simulink model "bibli_SM_R2023b_QUEVAL_20240121"  (R2023b)
settings: Solver=VariableStepAuto  StartTime=0.0  StopTime=10  MaxStep=1e-3  RelTol=1e-3
values from neighbouring files (symbols this model uses):
  Clark = [	2/3		-1/3		-1/3 ... (first row only)    [param_EESM.m]    (also in param_EESMdampers.m; param_PMSM.m)
  Fif = 0.259*3    (= 0.777)    [param_PMSM.m]
  InvClark = inv(Clark)    [param_EESM.m]    (also in param_EESMdampers.m; param_PMSM.m)
  INVL = inv(L)    [param_EESM.m]    (also in param_EESMdampers.m)
  J = 0.5    [param_EESM.m]    (also in param_EESMdampers.m; param_PMSM.m)
  Ld = 1.59e-2    (= 0.0159)    [param_EESM.m]    (also in param_EESMdampers.m; param_PMSM.m)
  Lq = 1.59e-2    (= 0.0159)    [param_EESM.m]    (also in param_EESMdampers.m; param_PMSM.m)
  M = [     0	    0	    -1 ... (first row only)    [param_EESM.m]    (also in param_EESMdampers.m = [     0	    0	    0	    -1	    0; param_PMSM.m = [     0	    -1)
  npp = 2    [param_EESM.m]    (also in param_EESMdampers.m; param_PMSM.m)
  R = [     Rs	    0	    0 ... (first row only)    [param_EESM.m]    (also in param_EESMdampers.m = [     Rs	    0	    0	    0	    0; param_PMSM.m = [     Rs	    0)
undefined symbols (not defined in the file or in its folder): fd, iao_pd_si, ibo_pd_si, ico_pd_si, Ts
libraries: spsSeriesRLCBranchLib x9, spsControlledCurrentSourceLib x9, spsVoltageMeasurementLib x9, spsControlledVoltageSourceLib x6, spsIdealSwitchLib x6, spsDCVoltageSourceLib x1, spsGroundLib x1, spspowerguiLib x1
(part 2 of 2)

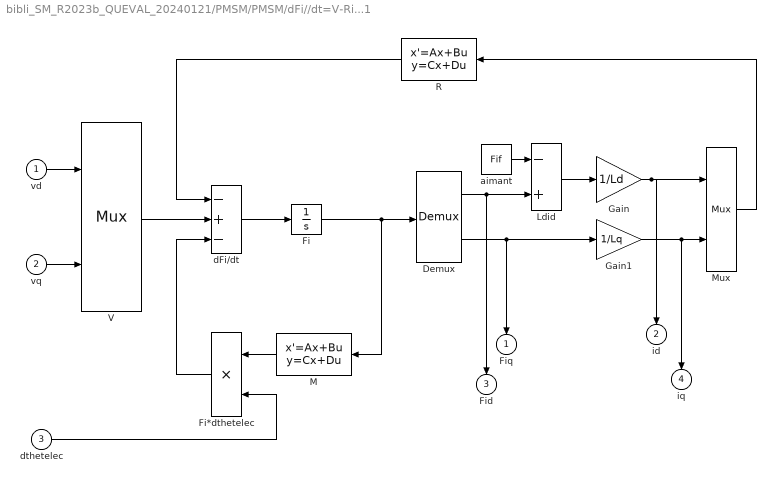
== system bibli_SM_R2023b_QUEVAL_20240121/PMSM/PMSM/dFi//dt=V-Ri...1 ==
  vd : Inport
  vq : Inport  Port=2
  dthetelec : Inport  Port=3
  Demux : Demux  Outputs=2
      settings: DisplayOption=none
  Fi : Integrator  InitialCondition=[Fif 0]
  Fi*dthetelec : Product  InputSameDT=on  SaturateOnIntegerOverflow=on  OutDataTypeStr=Inherit: Same as first input
  Gain : Gain  Gain=1/Ld  SaturateOnIntegerOverflow=on  OutDataTypeStr=Inherit: Same as input  ParamDataTypeStr=Inherit: Same as input
  Gain1 : Gain  Gain=1/Lq  SaturateOnIntegerOverflow=on  OutDataTypeStr=Inherit: Same as input  ParamDataTypeStr=Inherit: Same as input
  Ldid : Sum  Inputs=-+  InputSameDT=on  SaturateOnIntegerOverflow=on  OutDataTypeStr=Inherit: Same as first input
  M : StateSpace  A=[]  B=[]  C=[]  D=K  InitialCondition=0  mask(Matrix gain){K=M}
      mask prompts: K "Gain matrix:"
      mask help: Matrix Gain.
      mask Help: Multiplies input vector by entered matrix to produce output vector (y=Au).
      mask Display: disp('Matrice')
  Mux : Mux  Inputs=2
  R : StateSpace  A=[]  B=[]  C=[]  D=K  InitialCondition=0  mask(Matrix gain){K=R}
      mask prompts: K "Gain matrix:"
      mask help: Matrix Gain.
      mask Help: Multiplies input vector by entered matrix to produce output vector (y=Au).
      mask Display: disp('Matrice')
  V : Mux  Inputs=2
  aimant : Constant  Value=Fif
  dFi/dt : Sum  Inputs=-+-  InputSameDT=on  SaturateOnIntegerOverflow=on  OutDataTypeStr=Inherit: Same as first input
  Fiq : Outport  InitialOutput=0  VectorParamsAs1DForOutWhenUnconnected=off
  id : Outport  Port=2  InitialOutput=0  VectorParamsAs1DForOutWhenUnconnected=off
  Fid : Outport  Port=3  InitialOutput=0  VectorParamsAs1DForOutWhenUnconnected=off
  iq : Outport  Port=4  InitialOutput=0  VectorParamsAs1DForOutWhenUnconnected=off
  wires:
  Mux/1 -> R/1
  Gain1/1 -> iq/1, Mux/2
  Gain/1 -> id/1, Mux/1
  Demux/2 -> Fiq/1, Gain1/1
  Ldid/1 -> Gain/1
  aimant/1 -> Ldid/1
  Demux/1 -> Fid/1, Ldid/2
  Fi*dthetelec/1 -> dFi/dt/3
  M/1 -> Fi*dthetelec/1
  vq/1 -> V/2
  vd/1 -> V/1
  dFi/dt/1 -> Fi/1
  R/1 -> dFi/dt/1
  V/1 -> dFi/dt/2
  dthetelec/1 -> Fi*dthetelec/2
  Fi/1 -> Demux/1, M/1

== system bibli_SM_R2023b_QUEVAL_20240121/MS bobiné/MS bobiné/Park1/Clark ==
  a : Inport
  b : Inport  Port=2
  c : Inport  Port=3
  "Clark " : StateSpace  A=[]  B=[]  C=[]  D=K  InitialCondition=0  mask(Matrix Gain){K=Clark}
      mask prompts: K "Gain matrix:"
      mask help: Matrix Gain.
      mask Help: Multiplies input vector by entered matrix to produce output vector (y=Au).
      mask Display: disp('K')
  Demux : Demux  Outputs=3
      settings: DisplayOption=none
  Mux : Mux  Inputs=3
  alpha : Outport  InitialOutput=0  VectorParamsAs1DForOutWhenUnconnected=off
  beta : Outport  Port=2  InitialOutput=0  VectorParamsAs1DForOutWhenUnconnected=off
  o : Outport  Port=3  InitialOutput=0  VectorParamsAs1DForOutWhenUnconnected=off
  wires:
  Demux/3 -> o/1
  Demux/2 -> beta/1
  Demux/1 -> alpha/1
  "Clark "/1 -> Demux/1
  Mux/1 -> "Clark "/1
  c/1 -> Mux/3
  b/1 -> Mux/2
  a/1 -> Mux/1

== system bibli_SM_R2023b_QUEVAL_20240121/MS bobiné/MS bobiné/Park1/Rotation ==
  cos : Inport
  sin : Inport  Port=2
  alpha : Inport  Port=3
  beta : Inport  Port=4
  Product{,1..3} (4 alike) : Product  InputSameDT=on  RndMeth=Zero  SaturateOnIntegerOverflow=on  OutDataTypeStr=Inherit: Same as first input
  Sum : Sum  InputSameDT=on  SaturateOnIntegerOverflow=on  OutDataTypeStr=Inherit: Same as first input
  Sum1 : Sum  Inputs=-+  InputSameDT=on  SaturateOnIntegerOverflow=on  OutDataTypeStr=Inherit: Same as first input
  d : Outport  InitialOutput=0  VectorParamsAs1DForOutWhenUnconnected=off
  q : Outport  Port=2  InitialOutput=0  VectorParamsAs1DForOutWhenUnconnected=off
  wires:
  alpha/1 -> Product2/1, Product/2
  beta/1 -> Product3/2, Product1/2
  Sum1/1 -> q/1
  Sum/1 -> d/1
  Product3/1 -> Sum1/2
  Product2/1 -> Sum1/1
  cos/1 -> Product3/1, Product/1
  sin/1 -> Product2/2, Product1/1
  Product1/1 -> Sum/2
  Product/1 -> Sum/1

== system bibli_SM_R2023b_QUEVAL_20240121/MS bobiné/MS bobiné/Parkinv1/ClarkInv ==
  alpha : Inport
  beta : Inport  Port=2
  o : Inport  Port=3
  "ClarkInv " : StateSpace  A=[]  B=[]  C=[]  D=K  InitialCondition=0  mask(Matrix Gain){K=InvClark}
      mask prompts: K "Gain matrix:"
      mask help: Matrix Gain.
      mask Help: Multiplies input vector by entered matrix to produce output vector (y=Au).
      mask Display: disp('K')
  Demux : Demux  Outputs=3
      settings: DisplayOption=none
  Mux : Mux  Inputs=3
  a : Outport  InitialOutput=0  VectorParamsAs1DForOutWhenUnconnected=off
  b : Outport  Port=2  InitialOutput=0  VectorParamsAs1DForOutWhenUnconnected=off
  c : Outport  Port=3  InitialOutput=0  VectorParamsAs1DForOutWhenUnconnected=off
  wires:
  Demux/3 -> c/1
  Demux/2 -> b/1
  Demux/1 -> a/1
  "ClarkInv "/1 -> Demux/1
  Mux/1 -> "ClarkInv "/1
  o/1 -> Mux/3
  beta/1 -> Mux/2
  alpha/1 -> Mux/1

== system bibli_SM_R2023b_QUEVAL_20240121/MS bobiné/MS bobiné/Parkinv1/Rotation Inverse ==
  cos : Inport
  sin : Inport  Port=2
  d : Inport  Port=3
  q : Inport  Port=4
  Product{,1..3} (4 alike) : Product  InputSameDT=on  RndMeth=Zero  SaturateOnIntegerOverflow=on  OutDataTypeStr=Inherit: Same as first input
  Sum : Sum  Inputs=+-  InputSameDT=on  SaturateOnIntegerOverflow=on  OutDataTypeStr=Inherit: Same as first input
  Sum1 : Sum  InputSameDT=on  SaturateOnIntegerOverflow=on  OutDataTypeStr=Inherit: Same as first input
  alpha : Outport  InitialOutput=0  VectorParamsAs1DForOutWhenUnconnected=off
  beta : Outport  Port=2  InitialOutput=0  VectorParamsAs1DForOutWhenUnconnected=off
  wires:
  d/1 -> Product2/1, Product/2
  q/1 -> Product3/2, Product1/2
  Sum1/1 -> beta/1
  Sum/1 -> alpha/1
  Product3/1 -> Sum1/2
  Product2/1 -> Sum1/1
  cos/1 -> Product3/1, Product/1
  sin/1 -> Product2/2, Product1/1
  Product1/1 -> Sum/2
  Product/1 -> Sum/1

== system bibli_SM_R2023b_QUEVAL_20240121/MS bobiné amortisseurs/MS bobiné amortisseurs/Park/Clark ==
  a : Inport
  b : Inport  Port=2
  c : Inport  Port=3
  "Clark " : StateSpace  A=[]  B=[]  C=[]  D=K  InitialCondition=0  mask(Matrix Gain){K=Clark}
      mask prompts: K "Gain matrix:"
      mask help: Matrix Gain.
      mask Help: Multiplies input vector by entered matrix to produce output vector (y=Au).
      mask Display: disp('K')
  Demux : Demux  Outputs=3
      settings: DisplayOption=none
  Mux : Mux  Inputs=3
  alpha : Outport  InitialOutput=0  VectorParamsAs1DForOutWhenUnconnected=off
  beta : Outport  Port=2  InitialOutput=0  VectorParamsAs1DForOutWhenUnconnected=off
  o : Outport  Port=3  InitialOutput=0  VectorParamsAs1DForOutWhenUnconnected=off
  wires:
  Demux/3 -> o/1
  Demux/2 -> beta/1
  Demux/1 -> alpha/1
  "Clark "/1 -> Demux/1
  Mux/1 -> "Clark "/1
  c/1 -> Mux/3
  b/1 -> Mux/2
  a/1 -> Mux/1

== system bibli_SM_R2023b_QUEVAL_20240121/MS bobiné amortisseurs/MS bobiné amortisseurs/Park/Rotation ==
  cos : Inport
  sin : Inport  Port=2
  alpha : Inport  Port=3
  beta : Inport  Port=4
  Product{,1..3} (4 alike) : Product  InputSameDT=on  RndMeth=Zero  SaturateOnIntegerOverflow=on  OutDataTypeStr=Inherit: Same as first input
  Sum : Sum  InputSameDT=on  SaturateOnIntegerOverflow=on  OutDataTypeStr=Inherit: Same as first input
  Sum1 : Sum  Inputs=-+  InputSameDT=on  SaturateOnIntegerOverflow=on  OutDataTypeStr=Inherit: Same as first input
  d : Outport  InitialOutput=0  VectorParamsAs1DForOutWhenUnconnected=off
  q : Outport  Port=2  InitialOutput=0  VectorParamsAs1DForOutWhenUnconnected=off
  wires:
  alpha/1 -> Product2/1, Product/2
  beta/1 -> Product3/2, Product1/2
  Sum1/1 -> q/1
  Sum/1 -> d/1
  Product3/1 -> Sum1/2
  Product2/1 -> Sum1/1
  cos/1 -> Product3/1, Product/1
  sin/1 -> Product2/2, Product1/1
  Product1/1 -> Sum/2
  Product/1 -> Sum/1

== system bibli_SM_R2023b_QUEVAL_20240121/MS bobiné amortisseurs/MS bobiné amortisseurs/Parkinv/ClarkInv ==
  alpha : Inport
  beta : Inport  Port=2
  o : Inport  Port=3
  "ClarkInv " : StateSpace  A=[]  B=[]  C=[]  D=K  InitialCondition=0  mask(Matrix Gain){K=InvClark}
      mask prompts: K "Gain matrix:"
      mask help: Matrix Gain.
      mask Help: Multiplies input vector by entered matrix to produce output vector (y=Au).
      mask Display: disp('K')
  Demux : Demux  Outputs=3
      settings: DisplayOption=none
  Mux : Mux  Inputs=3
  a : Outport  InitialOutput=0  VectorParamsAs1DForOutWhenUnconnected=off
  b : Outport  Port=2  InitialOutput=0  VectorParamsAs1DForOutWhenUnconnected=off
  c : Outport  Port=3  InitialOutput=0  VectorParamsAs1DForOutWhenUnconnected=off
  wires:
  Demux/3 -> c/1
  Demux/2 -> b/1
  Demux/1 -> a/1
  "ClarkInv "/1 -> Demux/1
  Mux/1 -> "ClarkInv "/1
  o/1 -> Mux/3
  beta/1 -> Mux/2
  alpha/1 -> Mux/1

== system bibli_SM_R2023b_QUEVAL_20240121/MS bobiné amortisseurs/MS bobiné amortisseurs/Parkinv/Rotation Inverse ==
  cos : Inport
  sin : Inport  Port=2
  d : Inport  Port=3
  q : Inport  Port=4
  Product{,1..3} (4 alike) : Product  InputSameDT=on  RndMeth=Zero  SaturateOnIntegerOverflow=on  OutDataTypeStr=Inherit: Same as first input
  Sum : Sum  Inputs=+-  InputSameDT=on  SaturateOnIntegerOverflow=on  OutDataTypeStr=Inherit: Same as first input
  Sum1 : Sum  InputSameDT=on  SaturateOnIntegerOverflow=on  OutDataTypeStr=Inherit: Same as first input
  alpha : Outport  InitialOutput=0  VectorParamsAs1DForOutWhenUnconnected=off
  beta : Outport  Port=2  InitialOutput=0  VectorParamsAs1DForOutWhenUnconnected=off
  wires:
  d/1 -> Product2/1, Product/2
  q/1 -> Product3/2, Product1/2
  Sum1/1 -> beta/1
  Sum/1 -> alpha/1
  Product3/1 -> Sum1/2
  Product2/1 -> Sum1/1
  cos/1 -> Product3/1, Product/1
  sin/1 -> Product2/2, Product1/1
  Product1/1 -> Sum/2
  Product/1 -> Sum/1

== system bibli_SM_R2023b_QUEVAL_20240121/PMSM/PMSM/Park/Clark ==
  a : Inport
  b : Inport  Port=2
  c : Inport  Port=3
  "Clark " : StateSpace  A=[]  B=[]  C=[]  D=K  InitialCondition=0  mask(Matrix Gain){K=Clark}
      mask prompts: K "Gain matrix:"
      mask help: Matrix Gain.
      mask Help: Multiplies input vector by entered matrix to produce output vector (y=Au).
      mask Display: disp('K')
  Demux : Demux  Outputs=3
      settings: DisplayOption=none
  Mux : Mux  Inputs=3
  alpha : Outport  InitialOutput=0  VectorParamsAs1DForOutWhenUnconnected=off
  beta : Outport  Port=2  InitialOutput=0  VectorParamsAs1DForOutWhenUnconnected=off
  o : Outport  Port=3  InitialOutput=0  VectorParamsAs1DForOutWhenUnconnected=off
  wires:
  Demux/3 -> o/1
  Demux/2 -> beta/1
  Demux/1 -> alpha/1
  "Clark "/1 -> Demux/1
  Mux/1 -> "Clark "/1
  c/1 -> Mux/3
  b/1 -> Mux/2
  a/1 -> Mux/1

== system bibli_SM_R2023b_QUEVAL_20240121/PMSM/PMSM/Park/Rotation ==
  cos : Inport
  sin : Inport  Port=2
  alpha : Inport  Port=3
  beta : Inport  Port=4
  Product{,1..3} (4 alike) : Product  InputSameDT=on  SaturateOnIntegerOverflow=on  OutDataTypeStr=Inherit: Same as first input
  Sum : Sum  InputSameDT=on  SaturateOnIntegerOverflow=on  OutDataTypeStr=Inherit: Same as first input
  Sum1 : Sum  Inputs=-+  InputSameDT=on  SaturateOnIntegerOverflow=on  OutDataTypeStr=Inherit: Same as first input
  d : Outport  InitialOutput=0  VectorParamsAs1DForOutWhenUnconnected=off
  q : Outport  Port=2  InitialOutput=0  VectorParamsAs1DForOutWhenUnconnected=off
  wires:
  alpha/1 -> Product2/1, Product/2
  beta/1 -> Product3/2, Product1/2
  Sum1/1 -> q/1
  Sum/1 -> d/1
  Product3/1 -> Sum1/2
  Product2/1 -> Sum1/1
  cos/1 -> Product3/1, Product/1
  sin/1 -> Product2/2, Product1/1
  Product1/1 -> Sum/2
  Product/1 -> Sum/1

== system bibli_SM_R2023b_QUEVAL_20240121/PMSM/PMSM/Parkinv/ClarkInv ==
  alpha : Inport
  beta : Inport  Port=2
  o : Inport  Port=3
  "ClarkInv " : StateSpace  A=[]  B=[]  C=[]  D=K  InitialCondition=0  mask(Matrix Gain){K=InvClark}
      mask prompts: K "Gain matrix:"
      mask help: Matrix Gain.
      mask Help: Multiplies input vector by entered matrix to produce output vector (y=Au).
      mask Display: disp('K')
  Demux : Demux  Outputs=3
      settings: DisplayOption=none
  Mux : Mux  Inputs=3
  a : Outport  InitialOutput=0  VectorParamsAs1DForOutWhenUnconnected=off
  b : Outport  Port=2  InitialOutput=0  VectorParamsAs1DForOutWhenUnconnected=off
  c : Outport  Port=3  InitialOutput=0  VectorParamsAs1DForOutWhenUnconnected=off
  wires:
  Demux/3 -> c/1
  Demux/2 -> b/1
  Demux/1 -> a/1
  "ClarkInv "/1 -> Demux/1
  Mux/1 -> "ClarkInv "/1
  o/1 -> Mux/3
  beta/1 -> Mux/2
  alpha/1 -> Mux/1

== system bibli_SM_R2023b_QUEVAL_20240121/PMSM/PMSM/Parkinv/Rotation Inverse ==
  cos : Inport
  sin : Inport  Port=2
  d : Inport  Port=3
  q : Inport  Port=4
  Product{,1..3} (4 alike) : Product  InputSameDT=on  SaturateOnIntegerOverflow=on  OutDataTypeStr=Inherit: Same as first input
  Sum : Sum  Inputs=+-  InputSameDT=on  SaturateOnIntegerOverflow=on  OutDataTypeStr=Inherit: Same as first input
  Sum1 : Sum  InputSameDT=on  SaturateOnIntegerOverflow=on  OutDataTypeStr=Inherit: Same as first input
  alpha : Outport  InitialOutput=0  VectorParamsAs1DForOutWhenUnconnected=off
  beta : Outport  Port=2  InitialOutput=0  VectorParamsAs1DForOutWhenUnconnected=off
  wires:
  d/1 -> Product2/1, Product/2
  q/1 -> Product3/2, Product1/2
  Sum1/1 -> beta/1
  Sum/1 -> alpha/1
  Product3/1 -> Sum1/2
  Product2/1 -> Sum1/1
  cos/1 -> Product3/1, Product/1
  sin/1 -> Product2/2, Product1/1
  Product1/1 -> Sum/2
  Product/1 -> Sum/1
